simulink subsystem "Pacer"  (R2022a)
settings: Solver=VariableStepAuto  StartTime=0.0  StopTime=10.0  RelTol=1e-3
undefined symbols (not defined in the file): D10, D11, D12, D2, D4, D5, D7, D8, D9, PTA0, PTA2, PTB23, PTB9, PTC3, PTC4, PTD0, PTD2, PTD3
libraries: frdmk64flib x9, simulink x2
settings Model: Creator=bkfre  LastModifiedBy=bkfre

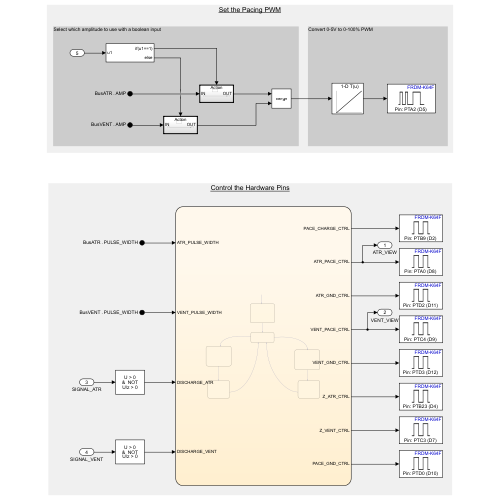
[thumbnail: Simulink's stored preview of the top-level diagram]
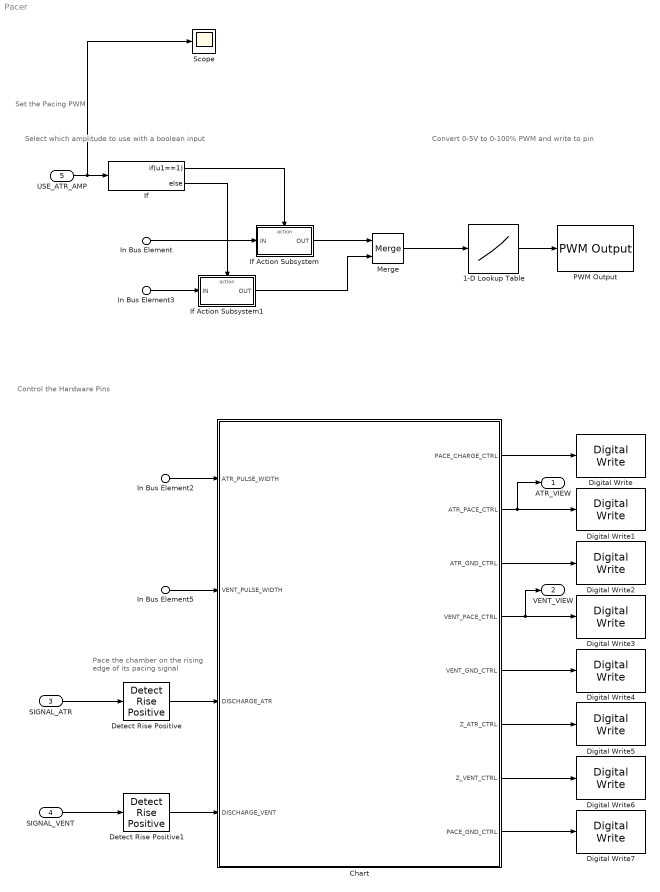
== system Pacer ==
  note: Pace the chamber on the rising edge of its pacing signal
  note: Control the Hardware Pins
  note: Convert 0-5V to 0-100% PWM and write to pin
  note: Select which amplitude to use with a boolean input
  note: Set the Pacing PWM
  In Bus Element : Inport  PortName=BusATR  Element=AMP
  In Bus Element2 : Inport  PortName=BusATR  Element=PULSE_WIDTH
  In Bus Element3 : Inport  Port=2  PortName=BusVENT  Element=AMP
  In Bus Element5 : Inport  Port=2  PortName=BusVENT  Element=PULSE_WIDTH
  SIGNAL_ATR : Inport  Port=3
  SIGNAL_VENT : Inport  Port=4
  USE_ATR_AMP : Inport  Port=5  OutDataTypeStr=boolean
  1-D Lookup Table : Lookup_n-D  NumberOfTableDimensions=1  BreakpointsForDimension1=[0,5]  Table=[0,100]  InternalRulePriority=Speed  RndMeth=Simplest
  Chart : Stateflow chart  TreatAsAtomicUnit=on
  Detect Rise Positive : simulink/Logic and Bit Operations/Detect Rise Positive  vinit=0  OutDataTypeStr=boolean
  Detect Rise Positive1 : simulink/Logic and Bit Operations/Detect Rise Positive  vinit=0  OutDataTypeStr=boolean
  Digital Write : frdmk64flib/Digital Write  Whichpin=PTB9 (D2)
  Digital Write1 : frdmk64flib/Digital Write  Whichpin=PTA0 (D8)
  Digital Write2 : frdmk64flib/Digital Write  Whichpin=PTD2 (D11)
  Digital Write3 : frdmk64flib/Digital Write  Whichpin=PTC4 (D9)
  Digital Write4 : frdmk64flib/Digital Write  Whichpin=PTD3 (D12)
  Digital Write5 : frdmk64flib/Digital Write  Whichpin=PTB23 (D4)
  Digital Write6 : frdmk64flib/Digital Write  Whichpin=PTC3 (D7)
  Digital Write7 : frdmk64flib/Digital Write  Whichpin=PTD0 (D10)
  If : If  IfExpression=u1==1
  If Action Subsystem : Subsystem  TreatAsAtomicUnit=on
  If Action Subsystem1 : Subsystem  TreatAsAtomicUnit=on
  Merge : Merge
  PWM Output : frdmk64flib/PWM Output  Whichpin=PTA2 (D5)  InitialFrequency=2000  InitialDutyCycle=100
  Scope : Scope
  ATR_VIEW : Outport
  VENT_VIEW : Outport  Port=2
  wires:
  Chart/1(PACE_CHARGE_CTRL) -> Digital Write/1
  Chart/2(ATR_PACE_CTRL) -> ATR_VIEW/1, Digital Write1/1
  Chart/3(ATR_GND_CTRL) -> Digital Write2/1
  Chart/4(VENT_PACE_CTRL) -> VENT_VIEW/1, Digital Write3/1
  Chart/5(VENT_GND_CTRL) -> Digital Write4/1
  Chart/6(Z_ATR_CTRL) -> Digital Write5/1
  Chart/7(Z_VENT_CTRL) -> Digital Write6/1
  Chart/8(PACE_GND_CTRL) -> Digital Write7/1
  In Bus Element5/1 -> Chart/2(VENT_PULSE_WIDTH)
  USE_ATR_AMP/1 -> If/1, Scope/1
  In Bus Element/1 -> If Action Subsystem/1(IN)
  If Action Subsystem/1(OUT) -> Merge/1
  If/2 -> If Action Subsystem1/Action
  If Action Subsystem1/1(OUT) -> Merge/2
  In Bus Element3/1 -> If Action Subsystem1/1(IN)
  If/1 -> If Action Subsystem/Action
  1-D Lookup Table/1 -> PWM Output/1
  Merge/1 -> 1-D Lookup Table/1
  SIGNAL_ATR/1 -> Detect Rise Positive/1
  SIGNAL_VENT/1 -> Detect Rise Positive1/1
  In Bus Element2/1 -> Chart/1(ATR_PULSE_WIDTH)
  Detect Rise Positive/1 -> Chart/3(DISCHARGE_ATR)
  Detect Rise Positive1/1 -> Chart/4(DISCHARGE_VENT)

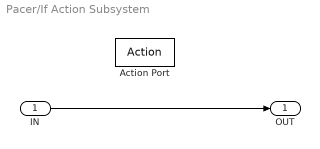
== system Pacer/If Action Subsystem ==
  IN : Inport
  Action Port : ActionPort
  OUT : Outport
  wires:
  IN/1 -> OUT/1

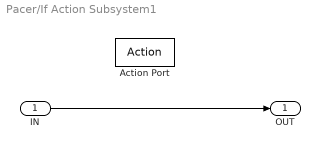
== system Pacer/If Action Subsystem1 ==
  IN : Inport
  Action Port : ActionPort
  OUT : Outport
  wires:
  IN/1 -> OUT/1

== stateflow chart Pacer/Chart ==
  settings: executeAtInitialization=1
  state Initialize
    entry:
    PACE_GND_CTRL=true;
    ATR_PACE_CTRL=false;
    VENT_PACE_CTRL=false;
    Z_ATR_CTRL=false;
    Z_VENT_CTRL=false;
    ATR_GND_CTRL=false;
    VENT_GND_CTRL=false;
    PACE_CHARGE_CTRL=true;
  state Charge
    entry:
    ATR_PACE_CTRL=false;
    VENT_PACE_CTRL=false;
    PACE_CHARGE_CTRL=true;
  state Discharge_ATR1
    entry:
    PACE_CHARGE_CTRL=false;
    PACE_GND_CTRL=true;
    VENT_PACE_CTRL=false;
    VENT_GND_CTRL=false;
    Z_VENT_CTRL=false;
    Z_ATR_CTRL=false;
    ATR_GND_CTRL=false;
    ATR_PACE_CTRL=true;
  state Discharge_VENT
    entry:
    PACE_CHARGE_CTRL=false;
    PACE_GND_CTRL=true;
    ATR_PACE_CTRL=false;
    ATR_GND_CTRL=false;
    Z_ATR_CTRL=false;
    Z_VENT_CTRL=false;
    VENT_GND_CTRL=false;
    VENT_PACE_CTRL=true;
  state Discharge_Blocking_ATR
    entry:
    PACE_GND_CTRL=true;
    ATR_PACE_CTRL=false;
    Z_VENT_CTRL=false;
    Z_ATR_CTRL=false;
    VENT_PACE_CTRL=false;
    VENT_GND_CTRL=false;
    ATR_GND_CTRL=true;
  state Discharge_Blocking_VENT
    entry:
    PACE_GND_CTRL=true;
    VENT_PACE_CTRL=false;
    Z_ATR_CTRL=false;
    Z_VENT_CTRL=false;
    ATR_PACE_CTRL=false;
    ATR_GND_CTRL=false;
    VENT_GND_CTRL=true;
  (default) -> Initialize
  Initialize -> Charge
  Charge -> Discharge_ATR1 [order 2] : [DISCHARGE_ATR>0]
  Charge -> Discharge_VENT [order 1] : [DISCHARGE_VENT>0]
  Discharge_Blocking_ATR -> Charge
  Discharge_Blocking_VENT -> Charge
  Discharge_ATR1 -> Discharge_Blocking_ATR : after(ATR_PULSE_WIDTH,msec)
  Discharge_VENT -> Discharge_Blocking_VENT : after(VENT_PULSE_WIDTH,msec)
  data: PACE_CHARGE_CTRL output boolean; ATR_PACE_CTRL output boolean; ATR_GND_CTRL output boolean; VENT_PACE_CTRL output boolean; VENT_GND_CTRL output boolean; Z_ATR_CTRL output boolean; Z_VENT_CTRL output boolean; PACE_GND_CTRL output boolean; ATR_PULSE_WIDTH input; VENT_PULSE_WIDTH input; DISCHARGE_ATR input boolean; DISCHARGE_VENT input boolean
